simulink model "gm_wlanhdlTimeAndFrequencySynchronization"  (R2025a)
settings: Solver=FixedStepDiscrete  StartTime=0.0  StopTime=stopTime  RelTol=1e-3
InitFcn:
  | wlanFrontEndInit;
undefined symbols (not defined in the file or in its folder): a, b, c, Hd, wlanConfig
libraries: simulink x95, hdlsllib x16, hdlmdlgenlib x12, dspsrcs4 x3, dspsigops x3, dsphdlsigops2 x2, dsphdlfiltering2 x2
(part 11 of 11)

== system gm_wlanhdlTimeAndFrequencySynchronization/WLANTimeAndFrequencySynchronization/Coarse Time Sync/Energy Calculator/magnitudeSquared/MagnitudeSquared ==
  dataIn : Inport  OutDataTypeStr=fixdt(1, 16, 12)  PortDimensions=1  SampleTime=5e-08
      settings: SignalType=complex
  validIn : Inport  Port=2  OutDataTypeStr=boolean  PortDimensions=1  SampleTime=5e-08
  Add : Sum  OutDataTypeStr=fixdt(1, 33, 24)  AccumDataTypeStr=fixdt(1, 33, 24)  SampleTime=6.25e-09
  Complex to Real-Imag : ComplexToRealImag  SampleTime=5e-08
  DTadjust : Subsystem
  Delay1 : Delay  DelayLength=double(2)  InitialCondition=0  SampleTime=5e-08
  Delay3 : Delay  DelayLength=double(2)  InitialCondition=0  SampleTime=5e-08
  Delay4 : RateTransition  InitialCondition=double(0)  OutPortSampleTimeOpt=Multiple of input port sample time  OutPortSampleTimeMultiple=8
  Delay4_absorbed : Delay  DelayLength=0
  Delay5 : RateTransition  InitialCondition=double(0)  OutPortSampleTimeOpt=Multiple of input port sample time  OutPortSampleTimeMultiple=8
  Delay5_absorbed : Delay  DelayLength=0
  Delay6 : Delay  DelayLength=double(2)  InitialCondition=0  SampleTime=5e-08
  Delay61 : RateTransition  InitialCondition=double(0)  OutPortSampleTimeOpt=Multiple of input port sample time  OutPortSampleTimeMultiple=8
  HwModeRegister{,1..3} (4 alike) : Delay  DelayLength=double(1)  InitialCondition=0  SampleTime=6.25e-09
  PipelineRegister : Delay  DelayLength=double(1)  InitialCondition=0  SampleTime=6.25e-09
  PipelineRegister1 : Delay  DelayLength=double(1)  InitialCondition=0  SampleTime=6.25e-09
  Product1 : Product  Inputs=**  OutDataTypeStr=fixdt(1, 32, 24)  SampleTime=6.25e-09
  Product4 : Product  Inputs=**  OutDataTypeStr=fixdt(1, 32, 24)  SampleTime=6.25e-09
  crp_out_delay : Delay  DelayLength=double(1)  InitialCondition=0  SampleTime=6.25e-09
  crp_out_delay1 : Delay  DelayLength=double(1)  InitialCondition=0  SampleTime=6.25e-09
  crp_out_delay2 : Delay  DelayLength=double(1)  InitialCondition=0  SampleTime=6.25e-09
  in0_repeat : RateTransition  Integrity=off  Deterministic=off  OutPortSampleTimeOpt=Multiple of input port sample time  OutPortSampleTimeMultiple=1/8
  in0_repeat1 : RateTransition  Integrity=off  Deterministic=off  OutPortSampleTimeOpt=Multiple of input port sample time  OutPortSampleTimeMultiple=1/8
  in1_repeat : RateTransition  Integrity=off  Deterministic=off  OutPortSampleTimeOpt=Multiple of input port sample time  OutPortSampleTimeMultiple=1/8
  in1_repeat1 : RateTransition  Integrity=off  Deterministic=off  OutPortSampleTimeOpt=Multiple of input port sample time  OutPortSampleTimeMultiple=1/8
  in2_repeat : RateTransition  Integrity=off  Deterministic=off  OutPortSampleTimeOpt=Multiple of input port sample time  OutPortSampleTimeMultiple=1/8
  in2_repeat1 : RateTransition  Integrity=off  Deterministic=off  OutPortSampleTimeOpt=Multiple of input port sample time  OutPortSampleTimeMultiple=1/8
  in3_repeat : RateTransition  Integrity=off  Deterministic=off  OutPortSampleTimeOpt=Multiple of input port sample time  OutPortSampleTimeMultiple=1/8
  rd_{0..4,11} (6 alike) : Delay  DelayLength=double(1)  InitialCondition=0  SampleTime=6.25e-09
  dataOut : Outport  SampleTime=6.25e-09  VectorParamsAs1DForOutWhenUnconnected=off
  validOut : Outport  Port=2  SampleTime=5e-08  VectorParamsAs1DForOutWhenUnconnected=off
  wires:
  DTadjust/1(out) -> dataOut/1
  rd_2/1 -> Add/2
  rd_1/1 -> Add/1
  in1_repeat/1 -> rd_1/1
  Delay5_absorbed/1 -> in2_repeat/1
  Delay4_absorbed/1 -> in1_repeat/1
  in3_repeat/1 -> rd_4/1
  in2_repeat/1 -> rd_2/1
  Delay61/1 -> Delay6/1
  in1_repeat1/1 -> rd_11/1
  rd_3/1 -> HwModeRegister2/1
  in0_repeat1/1 -> rd_0/1
  crp_out_delay/1 -> Delay61/1
  dataIn/1 -> Complex to Real-Imag/1
  Complex to Real-Imag/2 -> Delay3/1
  rd_4/1 -> HwModeRegister3/1
  Delay4/1 -> Delay4_absorbed/1
  rd_0/1 -> HwModeRegister/1
  validIn/1 -> in0_repeat/1
  Delay1/1 -> in1_repeat1/1, in0_repeat1/1
  HwModeRegister/1 -> Product4/1
  Product1/1 -> PipelineRegister1/1
  in0_repeat/1 -> crp_out_delay/1
  Delay6/1 -> validOut/1
  Complex to Real-Imag/1 -> Delay1/1
  rd_11/1 -> HwModeRegister1/1
  HwModeRegister1/1 -> Product4/2
  HwModeRegister2/1 -> Product1/1
  HwModeRegister3/1 -> Product1/2
  Delay3/1 -> in2_repeat1/1, in3_repeat/1
  Product4/1 -> PipelineRegister/1
  PipelineRegister/1 -> crp_out_delay1/1
  Delay5/1 -> Delay5_absorbed/1
  in2_repeat1/1 -> rd_3/1
  crp_out_delay2/1 -> Delay5/1
  PipelineRegister1/1 -> crp_out_delay2/1
  Add/1 -> DTadjust/1(in)
  crp_out_delay1/1 -> Delay4/1

== system gm_wlanhdlTimeAndFrequencySynchronization/WLANTimeAndFrequencySynchronization/Coarse Time Sync/Energy Calculator/magnitudeSquared/MagnitudeSquared1 ==
  dataIn : Inport  OutDataTypeStr=fixdt(1, 35, 27)  PortDimensions=1  SampleTime=6.25e-09
  validIn : Inport  Port=2  OutDataTypeStr=boolean  PortDimensions=1  SampleTime=5e-08
  Add : Sum  OutDataTypeStr=fixdt(1, 71, 54)  AccumDataTypeStr=fixdt(1, 71, 54)  SampleTime=6.25e-09
  Complex to Real-Imag : ComplexToRealImag  SampleTime=6.25e-09
  Delay{,1..3} (4 alike) : Delay  DelayLength=double(1)  InitialCondition=0  SampleTime=5e-08
  Delay{4..5,11,21,31,41,61} (7 alike) : RateTransition  InitialCondition=double(0)  OutPortSampleTimeOpt=Multiple of input port sample time  OutPortSampleTimeMultiple=8
  Delay4_absorbed : Delay  DelayLength=0
  Delay5_absorbed : Delay  DelayLength=0
  Delay6 : Delay  DelayLength=double(3)  InitialCondition=0  SampleTime=5e-08
  HwModeRegister{,1..3} (4 alike) : Delay  DelayLength=double(1)  InitialCondition=0  SampleTime=6.25e-09
  PipelineRegister : Delay  DelayLength=double(1)  InitialCondition=0  SampleTime=6.25e-09
  PipelineRegister1 : Delay  DelayLength=double(1)  InitialCondition=0  SampleTime=6.25e-09
  Product1 : Product  Inputs=**  OutDataTypeStr=fixdt(1, 70, 54)  SampleTime=6.25e-09
  Product4 : Product  Inputs=**  OutDataTypeStr=fixdt(1, 70, 54)  SampleTime=6.25e-09
  crp_out_delay{,1..3} (4 alike) : Delay  DelayLength=double(1)  InitialCondition=0  SampleTime=6.25e-09
  in0_repeat : RateTransition  Integrity=off  Deterministic=off  OutPortSampleTimeOpt=Multiple of input port sample time  OutPortSampleTimeMultiple=1/8
  in0_repeat1 : RateTransition  Integrity=off  Deterministic=off  OutPortSampleTimeOpt=Multiple of input port sample time  OutPortSampleTimeMultiple=1/8
  in1_repeat : RateTransition  Integrity=off  Deterministic=off  OutPortSampleTimeOpt=Multiple of input port sample time  OutPortSampleTimeMultiple=1/8
  in1_repeat1 : RateTransition  Integrity=off  Deterministic=off  OutPortSampleTimeOpt=Multiple of input port sample time  OutPortSampleTimeMultiple=1/8
  in2_repeat : RateTransition  Integrity=off  Deterministic=off  OutPortSampleTimeOpt=Multiple of input port sample time  OutPortSampleTimeMultiple=1/8
  in2_repeat1 : RateTransition  Integrity=off  Deterministic=off  OutPortSampleTimeOpt=Multiple of input port sample time  OutPortSampleTimeMultiple=1/8
  in3_repeat : RateTransition  Integrity=off  Deterministic=off  OutPortSampleTimeOpt=Multiple of input port sample time  OutPortSampleTimeMultiple=1/8
  rd_{0..4,11} (6 alike) : Delay  DelayLength=double(1)  InitialCondition=0  SampleTime=6.25e-09
  dataOut : Outport  SampleTime=6.25e-09  VectorParamsAs1DForOutWhenUnconnected=off
  validOut : Outport  Port=2  SampleTime=5e-08  VectorParamsAs1DForOutWhenUnconnected=off
  wires:
  rd_2/1 -> Add/2
  in2_repeat/1 -> rd_2/1
  in1_repeat/1 -> rd_1/1
  Delay5_absorbed/1 -> in2_repeat/1
  Delay4_absorbed/1 -> in1_repeat/1
  crp_out_delay1/1 -> Delay5/1
  crp_out_delay/1 -> Delay41/1
  PipelineRegister1/1 -> crp_out_delay1/1
  PipelineRegister/1 -> crp_out_delay/1
  Delay31/1 -> Delay3/1
  in0_repeat/1 -> Delay61/1
  Delay11/1 -> Delay1/1
  HwModeRegister1/1 -> Product4/2
  crp_out_delay3/1 -> Delay21/1, Delay31/1
  Delay5/1 -> Delay5_absorbed/1
  crp_out_delay2/1 -> Delay4/1, Delay11/1
  Delay21/1 -> Delay2/1
  Delay61/1 -> Delay6/1
  HwModeRegister2/1 -> Product1/1
  Complex to Real-Imag/2 -> crp_out_delay3/1
  Product4/1 -> PipelineRegister/1
  Complex to Real-Imag/1 -> crp_out_delay2/1
  Delay4/1 -> Delay/1
  rd_3/1 -> HwModeRegister2/1
  Delay6/1 -> validOut/1
  Delay41/1 -> Delay4_absorbed/1
  rd_11/1 -> HwModeRegister1/1
  rd_1/1 -> Add/1
  validIn/1 -> in0_repeat/1
  rd_4/1 -> HwModeRegister3/1
  Delay3/1 -> in3_repeat/1
  dataIn/1 -> Complex to Real-Imag/1
  Delay/1 -> in1_repeat1/1
  Delay2/1 -> in2_repeat1/1
  Product1/1 -> PipelineRegister1/1
  in0_repeat1/1 -> rd_0/1
  Delay1/1 -> in0_repeat1/1
  in1_repeat1/1 -> rd_11/1
  in3_repeat/1 -> rd_4/1
  Add/1 -> dataOut/1
  rd_0/1 -> HwModeRegister/1
  in2_repeat1/1 -> rd_3/1
  HwModeRegister/1 -> Product4/1
  HwModeRegister3/1 -> Product1/2

== system gm_wlanhdlTimeAndFrequencySynchronization/WLANTimeAndFrequencySynchronization/Coarse Time Sync/Energy Calculator/magnitudeSquared/MovingSum ==
  dataIn : Inport  OutDataTypeStr=fixdt(1, 34, 27)  PortDimensions=1  SampleTime=6.25e-09
  validIn : Inport  Port=2  OutDataTypeStr=boolean  PortDimensions=1  SampleTime=5e-08
  Add : Sum  Inputs=+-  OutDataTypeStr=fixdt(1, 35, 27)  AccumDataTypeStr=fixdt(1, 35, 27)  SampleTime=6.25e-09
  Add1 : Sum  OutDataTypeStr=fixdt(1, 35, 27)  AccumDataTypeStr=fixdt(1, 35, 27)  SampleTime=6.25e-09
  Delay12 : RateTransition  InitialCondition=double(0)  OutPortSampleTimeOpt=Multiple of input port sample time  OutPortSampleTimeMultiple=8
  Delay12_absorbed : Delay  DelayLength=0
  Delay{3..6} (4 alike) : Delay  DelayLength=double(1)  InitialCondition=0  SampleTime=5e-08
  Delay31 : RateTransition  InitialCondition=double(0)  OutPortSampleTimeOpt=Multiple of input port sample time  OutPortSampleTimeMultiple=8
  Delay41 : RateTransition  InitialCondition=double(0)  OutPortSampleTimeOpt=Multiple of input port sample time  OutPortSampleTimeMultiple=8
  Delay_Switch : Switch  Criteria=u2 ~= 0  Threshold=double(0)  OutDataTypeStr=fixdt(1, 35, 27)  SampleTime=6.25e-09  SaturateOnIntegerOverflow=off  InputSameDT=off
  Shift Arithmetic : ArithShift  BitShiftNumber=double(1)  BinPtShiftNumber=double(0)
  "Synchronous Enabled 16 Sample Delay " : Subsystem
  Synchronous Enabled Unit Delay_lowered : RateTransition  InitialCondition=double(0)  OutPortSampleTimeOpt=Multiple of input port sample time  OutPortSampleTimeMultiple=8
  Synchronous Enabled Unit Delay_lowered_absorbed : Delay  DelayLength=0
  crp_out_delay : Delay  DelayLength=double(1)  InitialCondition=0  SampleTime=6.25e-09
  crp_out_delay1 : Delay  DelayLength=double(1)  InitialCondition=0  SampleTime=6.25e-09
  in0_repeat : RateTransition  Integrity=off  Deterministic=off  OutPortSampleTimeOpt=Multiple of input port sample time  OutPortSampleTimeMultiple=1/8
  in0_repeat1 : RateTransition  Integrity=off  Deterministic=off  OutPortSampleTimeOpt=Multiple of input port sample time  OutPortSampleTimeMultiple=1/8
  in1_repeat : RateTransition  Integrity=off  Deterministic=off  OutPortSampleTimeOpt=Multiple of input port sample time  OutPortSampleTimeMultiple=1/8
  in2_repeat : RateTransition  Integrity=off  Deterministic=off  OutPortSampleTimeOpt=Multiple of input port sample time  OutPortSampleTimeMultiple=1/8
  in2_repeat1 : RateTransition  Integrity=off  Deterministic=off  OutPortSampleTimeOpt=Multiple of input port sample time  OutPortSampleTimeMultiple=1/8
  rd_{1,3,5,11,21,31} (6 alike) : Delay  DelayLength=double(1)  InitialCondition=0  SampleTime=6.25e-09
  rd_2 : Delay  DelayLength=double(3)  InitialCondition=0  SampleTime=6.25e-09
  rd_4 : Delay  DelayLength=double(2)  InitialCondition=0  SampleTime=6.25e-09
  dataOut : Outport  SampleTime=5e-08  VectorParamsAs1DForOutWhenUnconnected=off
  validOut : Outport  Port=2  SampleTime=5e-08  VectorParamsAs1DForOutWhenUnconnected=off
  wires:
  rd_21/1 -> Add1/2, rd_5/1
  rd_11/1 -> Add1/1
  Delay41/1 -> Delay4/1
  Delay6/1 -> validOut/1
  in0_repeat1/1 -> Delay41/1, rd_4/1
  rd_2/1 -> Add/2
  in1_repeat/1 -> rd_21/1
  Delay3/1 -> in0_repeat1/1
  in2_repeat/1 -> rd_2/1
  rd_1/1 -> Add/1
  Delay31/1 -> Delay3/1
  dataIn/1 -> "Synchronous Enabled 16 Sample Delay "/1(dataIn), rd_1/1
  in0_repeat/1 -> Delay31/1
  rd_3/1 -> Shift Arithmetic/1
  "Synchronous Enabled 16 Sample Delay "/1(dataOut) -> in2_repeat/1
  validIn/1 -> "Synchronous Enabled 16 Sample Delay "/2(en), in0_repeat/1
  Synchronous Enabled Unit Delay_lowered_absorbed/1 -> in1_repeat/1, Delay5/1
  rd_5/1 -> Delay_Switch/3
  rd_4/1 -> Delay_Switch/2
  crp_out_delay/1 -> Delay12/1
  crp_out_delay1/1 -> Synchronous Enabled Unit Delay_lowered/1
  Synchronous Enabled Unit Delay_lowered/1 -> Synchronous Enabled Unit Delay_lowered_absorbed/1
  rd_31/1 -> Delay_Switch/1
  Delay4/1 -> Delay6/1
  Shift Arithmetic/1 -> crp_out_delay/1
  Delay_Switch/1 -> crp_out_delay1/1
  Add1/1 -> rd_31/1
  Add/1 -> rd_3/1
  Delay12/1 -> Delay12_absorbed/1
  in2_repeat1/1 -> rd_11/1
  Delay12_absorbed/1 -> in2_repeat1/1
  Delay5/1 -> dataOut/1

== system gm_wlanhdlTimeAndFrequencySynchronization/WLANTimeAndFrequencySynchronization/Coarse Time Sync/Energy Calculator/streamSynchronizer/StreamSyncronizer ==
  pop : Inport  OutDataTypeStr=boolean  PortDimensions=1  SampleTime=5e-08
  dataIn : Inport  Port=2  OutDataTypeStr=fixdt(1, 71, 54)  PortDimensions=1  SampleTime=5e-08
  push : Inport  Port=3  OutDataTypeStr=boolean  PortDimensions=1  SampleTime=5e-08
  StreamSyncronizer : MATLAB Function  InitFcn=Simulink.suppressDiagnostic(gcb, 'Stateflow:Runtime:DataOverflowErrorMSLD');  TreatAsAtomicUnit=on  mask{depth=256}
      mask help: Synchronize two data streams with a FIFO.
  dataOut : Outport  SampleTime=5e-08  VectorParamsAs1DForOutWhenUnconnected=off
  validOut : Outport  Port=2  SampleTime=5e-08  VectorParamsAs1DForOutWhenUnconnected=off
  wires:
  StreamSyncronizer/2(validOut) -> validOut/1
  StreamSyncronizer/1(dataOut) -> dataOut/1
  push/1 -> StreamSyncronizer/3(push)
  dataIn/1 -> StreamSyncronizer/2(dataIn)
  pop/1 -> StreamSyncronizer/1(pop)

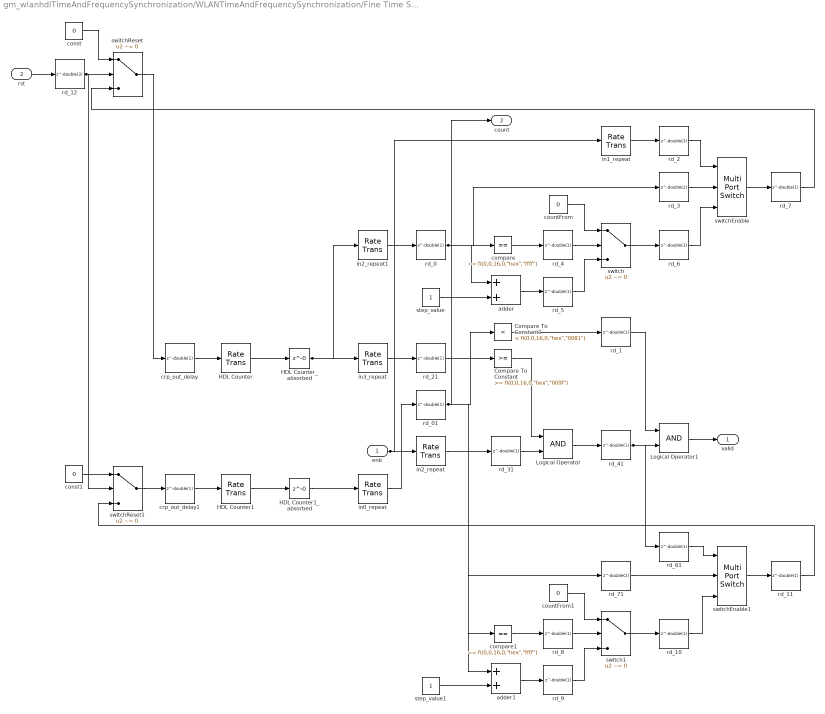
== system gm_wlanhdlTimeAndFrequencySynchronization/WLANTimeAndFrequencySynchronization/Fine Time Sync/Peak Searcher/maxPeakSearcher/extractLTFs ==
  enb : Inport  OutDataTypeStr=boolean  PortDimensions=1  SampleTime=5e-08
  rst : Inport  Port=2  OutDataTypeStr=boolean  PortDimensions=1  SampleTime=6.25e-09
  Compare To Constant : simulink/Logic and Bit Operations/Compare To Constant  relop=>=  const="fi(0,0,16,0,\"hex\",\"009f\")"  OutDataTypeStr=boolean
  Compare To Constant1 : simulink/Logic and Bit Operations/Compare To Constant  relop=<  const="fi(0,0,16,0,\"hex\",\"0081\")"  OutDataTypeStr=boolean
  HDL Counter : RateTransition  InitialCondition=double(0)  OutPortSampleTimeOpt=Multiple of input port sample time  OutPortSampleTimeMultiple=8
  HDL Counter1 : RateTransition  InitialCondition=double(0)  OutPortSampleTimeOpt=Multiple of input port sample time  OutPortSampleTimeMultiple=8
  HDL Counter1_absorbed : Delay  DelayLength=0
  HDL Counter_absorbed : Delay  DelayLength=0
  Logical Operator : Logic  AllPortsSameDT=off  OutDataTypeStr=boolean  SampleTime=6.25e-09
  Logical Operator1 : Logic  AllPortsSameDT=off  OutDataTypeStr=boolean  SampleTime=6.25e-09
  adder : Sum  OutDataTypeStr=uint16  AccumDataTypeStr=uint16  SampleTime=6.25e-09
  adder1 : Sum  OutDataTypeStr=uint16  AccumDataTypeStr=uint16  SampleTime=6.25e-09
  compare : simulink/Logic and Bit Operations/Compare To Constant  relop===  const="fi(0,0,16,0,\"hex\",\"ffff\")"  OutDataTypeStr=boolean
  compare1 : simulink/Logic and Bit Operations/Compare To Constant  relop===  const="fi(0,0,16,0,\"hex\",\"ffff\")"  OutDataTypeStr=boolean
  const : Constant  Value=0  VectorParams1D=off  OutDataTypeStr=uint16  SampleTime=6.25e-09
  const1 : Constant  Value=0  VectorParams1D=off  OutDataTypeStr=uint16  SampleTime=6.25e-09
  countFrom : Constant  Value=0  VectorParams1D=off  OutDataTypeStr=uint16  SampleTime=6.25e-09
  countFrom1 : Constant  Value=0  VectorParams1D=off  OutDataTypeStr=uint16  SampleTime=6.25e-09
  crp_out_delay : Delay  DelayLength=double(1)  InitialCondition=0  SampleTime=6.25e-09
  crp_out_delay1 : Delay  DelayLength=double(1)  InitialCondition=0  SampleTime=6.25e-09
  in0_repeat : RateTransition  Integrity=off  Deterministic=off  OutPortSampleTimeOpt=Multiple of input port sample time  OutPortSampleTimeMultiple=1/8
  in1_repeat : RateTransition  Integrity=off  Deterministic=off  OutPortSampleTimeOpt=Multiple of input port sample time  OutPortSampleTimeMultiple=1/8
  in2_repeat : RateTransition  Integrity=off  Deterministic=off  OutPortSampleTimeOpt=Multiple of input port sample time  OutPortSampleTimeMultiple=1/8
  in2_repeat1 : RateTransition  Integrity=off  Deterministic=off  OutPortSampleTimeOpt=Multiple of input port sample time  OutPortSampleTimeMultiple=1/8
  in3_repeat : RateTransition  Integrity=off  Deterministic=off  OutPortSampleTimeOpt=Multiple of input port sample time  OutPortSampleTimeMultiple=1/8
  rd_{0..1,4..11,21,31,41,61} (14 alike) : Delay  DelayLength=double(1)  InitialCondition=0  SampleTime=6.25e-09
  rd_01 : Delay  DelayLength=double(1)  InitialCondition=0  SampleTime=6.25e-09
  rd_12 : Delay  DelayLength=double(3)  InitialCondition=0  SampleTime=6.25e-09
  rd_2 : Delay  DelayLength=double(3)  InitialCondition=0  SampleTime=6.25e-09
  rd_3 : Delay  DelayLength=double(2)  InitialCondition=0  SampleTime=6.25e-09
  rd_71 : Delay  DelayLength=double(2)  InitialCondition=0  SampleTime=6.25e-09
  step_value : Constant  VectorParams1D=off  OutDataTypeStr=uint16  SampleTime=6.25e-09
  step_value1 : Constant  VectorParams1D=off  OutDataTypeStr=uint16  SampleTime=6.25e-09
  switch : Switch  Criteria=u2 ~= 0  Threshold="fi(0,0,1,0,\"hex\",\"0\")"  OutDataTypeStr=uint16  SampleTime=6.25e-09  SaturateOnIntegerOverflow=off  InputSameDT=off
  switch1 : Switch  Criteria=u2 ~= 0  Threshold="fi(0,0,1,0,\"hex\",\"0\")"  OutDataTypeStr=uint16  SampleTime=6.25e-09  SaturateOnIntegerOverflow=off  InputSameDT=off
  switchEnable : MultiPortSwitch  DataPortOrder=Zero-based contiguous  Inputs=2  DiagnosticForDefault=None  zeroidx=on  OutDataTypeStr=uint16  SampleTime=6.25e-09  SaturateOnIntegerOverflow=off  InputSameDT=off
  switchEnable1 : MultiPortSwitch  DataPortOrder=Zero-based contiguous  Inputs=2  DiagnosticForDefault=None  zeroidx=on  OutDataTypeStr=uint16  SampleTime=6.25e-09  SaturateOnIntegerOverflow=off  InputSameDT=off
  switchReset : Switch  Criteria=u2 ~= 0  Threshold="fi(0,0,1,0,\"hex\",\"0\")"  OutDataTypeStr=uint16  SampleTime=6.25e-09  SaturateOnIntegerOverflow=off  InputSameDT=off
  switchReset1 : Switch  Criteria=u2 ~= 0  Threshold="fi(0,0,1,0,\"hex\",\"0\")"  OutDataTypeStr=uint16  SampleTime=6.25e-09  SaturateOnIntegerOverflow=off  InputSameDT=off
  valid : Outport  SampleTime=6.25e-09
  count : Outport  Port=2  SampleTime=6.25e-09
  wires:
  rd_7/1 -> switchReset/3
  rd_10/1 -> switchEnable1/3
  rd_61/1 -> switchEnable1/1
  rd_6/1 -> switchEnable/3
  rd_71/1 -> switchEnable1/2
  rd_41/1 -> rd_61/1, Logical Operator1/2
  switch/1 -> rd_6/1
  countFrom1/1 -> switch1/1
  switchEnable1/1 -> rd_11/1
  Logical Operator/1 -> rd_41/1
  rd_11/1 -> switchReset1/3
  rd_5/1 -> switch/3
  rd_4/1 -> switch/2
  countFrom/1 -> switch/1
  rd_3/1 -> switchEnable/2
  HDL Counter1_absorbed/1 -> in0_repeat/1
  in1_repeat/1 -> rd_2/1
  in2_repeat/1 -> rd_31/1
  compare1/1 -> rd_8/1
  crp_out_delay1/1 -> HDL Counter1/1
  crp_out_delay/1 -> HDL Counter/1
  switchReset1/1 -> crp_out_delay1/1
  HDL Counter/1 -> HDL Counter_absorbed/1
  rd_31/1 -> Logical Operator/2
  const1/1 -> switchReset1/1
  HDL Counter_absorbed/1 -> in2_repeat1/1, in3_repeat/1
  rd_12/1 -> switchReset1/2, switchReset/2
  switchEnable/1 -> rd_7/1
  switchReset/1 -> crp_out_delay/1
  const/1 -> switchReset/1
  step_value/1 -> adder/2
  rd_9/1 -> switch1/3
  in3_repeat/1 -> rd_21/1
  enb/1 -> in2_repeat/1, in1_repeat/1
  Logical Operator1/1 -> valid/1
  in0_repeat/1 -> rd_01/1
  compare/1 -> rd_4/1
  rd_0/1 -> compare/1, adder/1, rd_3/1
  rd_21/1 -> Compare To Constant/1
  rst/1 -> rd_12/1
  rd_01/1 -> count/1, rd_71/1, Compare To Constant1/1, compare1/1, adder1/1
  switch1/1 -> rd_10/1
  step_value1/1 -> adder1/2
  Compare To Constant/1 -> Logical Operator/1
  HDL Counter1/1 -> HDL Counter1_absorbed/1
  adder/1 -> rd_5/1
  rd_2/1 -> switchEnable/1
  rd_1/1 -> Logical Operator1/1
  Compare To Constant1/1 -> rd_1/1
  rd_8/1 -> switch1/2
  in2_repeat1/1 -> rd_0/1
  adder1/1 -> rd_9/1

== system gm_wlanhdlTimeAndFrequencySynchronization/WLANTimeAndFrequencySynchronization/Fine Time Sync/Peak Searcher/maxPeakSearcher/maxPeakSearcher ==
  dataIn : Inport  OutDataTypeStr=fixdt(1, 32, 15)  PortDimensions=1  SampleTime=5e-08
  validIn : Inport  Port=2  OutDataTypeStr=boolean  PortDimensions=1  SampleTime=5e-08
  countValue : Inport  Port=3  OutDataTypeStr=uint16  PortDimensions=1  SampleTime=5e-08
  reset : Inport  Port=4  OutDataTypeStr=boolean  PortDimensions=1  SampleTime=5e-08
  maxPeakSearcher : MATLAB Function  TreatAsAtomicUnit=on
  maxPeak : Outport  SampleTime=5e-08  VectorParamsAs1DForOutWhenUnconnected=off
  wires:
  maxPeakSearcher/1(maxPeak) -> maxPeak/1
  reset/1 -> maxPeakSearcher/4(reset)
  countValue/1 -> maxPeakSearcher/3(countValue)
  validIn/1 -> maxPeakSearcher/2(validIn)
  dataIn/1 -> maxPeakSearcher/1(dataIn)

== system gm_wlanhdlTimeAndFrequencySynchronization/WLANTimeAndFrequencySynchronization/Fine Time Sync/Peak Searcher/peakDetector/dataSelector  ==
  syncEn : Inport  OutDataTypeStr=boolean  PortDimensions=1  SampleTime=5e-08
  dataIn : Inport  Port=2  OutDataTypeStr=fixdt(1, 16, 12)  PortDimensions=1  SampleTime=5e-08
      settings: SignalType=complex
  validIn : Inport  Port=3  OutDataTypeStr=boolean  PortDimensions=1  SampleTime=5e-08
  MATLAB Function1 : MATLAB Function  TreatAsAtomicUnit=on
  dataOut : Outport  SampleTime=5e-08  VectorParamsAs1DForOutWhenUnconnected=off
  wires:
  syncEn/1 -> MATLAB Function1/1(syncEn)
  dataIn/1 -> MATLAB Function1/2(dataIn)
  validIn/1 -> MATLAB Function1/3(validIn)
  MATLAB Function1/1(dataOut) -> dataOut/1

== system gm_wlanhdlTimeAndFrequencySynchronization/WLANTimeAndFrequencySynchronization/Coarse Time Sync/Energy Calculator/magnitudeSquared/MagnitudeSquared/DTadjust ==
  in : Inport  OutDataTypeStr=fixdt(1, 33, 24)  PortDimensions=1  SampleTime=6.25e-09
  DTadjust : MATLAB Function  TreatAsAtomicUnit=on
  out : Outport  SampleTime=6.25e-09  VectorParamsAs1DForOutWhenUnconnected=off
  wires:
  DTadjust/1(out) -> out/1
  in/1 -> DTadjust/1(in)

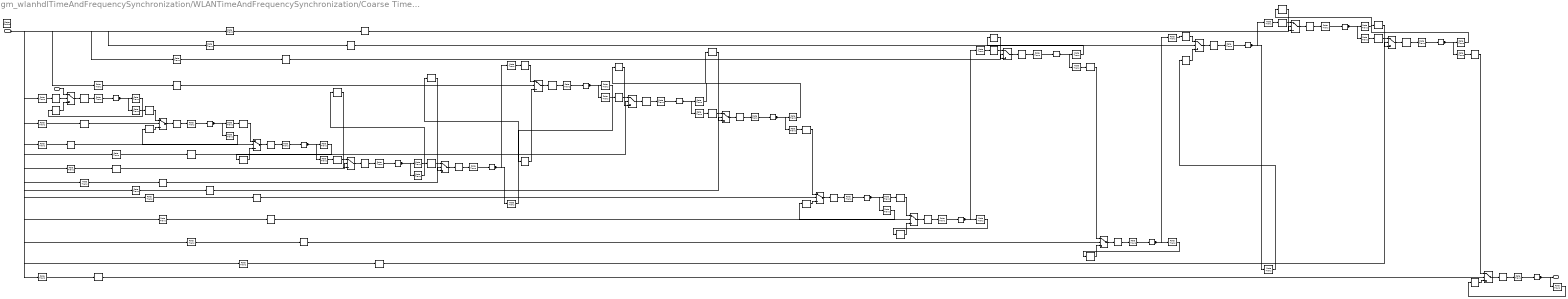
== system gm_wlanhdlTimeAndFrequencySynchronization/WLANTimeAndFrequencySynchronization/Coarse Time Sync/Energy Calculator/magnitudeSquared/MovingSum/Synchronous Enabled 16 Sample Delay  ==
  dataIn : Inport  OutDataTypeStr=fixdt(1, 34, 27)  PortDimensions=1  SampleTime=6.25e-09
  en : Inport  Port=2  OutDataTypeStr=boolean  PortDimensions=1  SampleTime=5e-08
  Delay1_lowered{,1..15} (16 alike) : RateTransition  InitialCondition=double(0)  OutPortSampleTimeOpt=Multiple of input port sample time  OutPortSampleTimeMultiple=8
  Delay1_lowered_absorbed{,1..15} (16 alike) : Delay  DelayLength=0
  Delay_Switch{,1..15} (16 alike) : Switch  Criteria=u2 ~= 0  Threshold=double(0)  OutDataTypeStr=fixdt(1, 34, 27)  SampleTime=6.25e-09  SaturateOnIntegerOverflow=off  InputSameDT=off
  StateControl : StateControl  StateControl=Synchronous
  crp_out_delay{,1..15} (16 alike) : Delay  DelayLength=double(1)  InitialCondition=0  SampleTime=6.25e-09
  in0_repeat{,1..14} (15 alike) : RateTransition  Integrity=off  Deterministic=off  OutPortSampleTimeOpt=Multiple of input port sample time  OutPortSampleTimeMultiple=1/8
  in1_repeat{,1..15} (16 alike) : RateTransition  Integrity=off  Deterministic=off  OutPortSampleTimeOpt=Multiple of input port sample time  OutPortSampleTimeMultiple=1/8
  in2_repeat{,1..15} (16 alike) : RateTransition  Integrity=off  Deterministic=off  OutPortSampleTimeOpt=Multiple of input port sample time  OutPortSampleTimeMultiple=1/8
  rd_0 : Delay  DelayLength=double(2)  InitialCondition=0  SampleTime=6.25e-09
  rd_01 : Delay  DelayLength=double(1)  InitialCondition=0  SampleTime=6.25e-09
  rd_010 : Delay  DelayLength=double(1)  InitialCondition=0  SampleTime=6.25e-09
  rd_011 : Delay  DelayLength=double(1)  InitialCondition=0  SampleTime=6.25e-09
  rd_012 : Delay  DelayLength=double(1)  InitialCondition=0  SampleTime=6.25e-09
  rd_013 : Delay  DelayLength=double(1)  InitialCondition=0  SampleTime=6.25e-09
  rd_014 : Delay  DelayLength=double(1)  InitialCondition=0  SampleTime=6.25e-09
  rd_015 : Delay  DelayLength=double(1)  InitialCondition=0  SampleTime=6.25e-09
  rd_02 : Delay  DelayLength=double(1)  InitialCondition=0  SampleTime=6.25e-09
  rd_03 : Delay  DelayLength=double(1)  InitialCondition=0  SampleTime=6.25e-09
  rd_04 : Delay  DelayLength=double(1)  InitialCondition=0  SampleTime=6.25e-09
  rd_05 : Delay  DelayLength=double(1)  InitialCondition=0  SampleTime=6.25e-09
  rd_06 : Delay  DelayLength=double(1)  InitialCondition=0  SampleTime=6.25e-09
  rd_07 : Delay  DelayLength=double(1)  InitialCondition=0  SampleTime=6.25e-09
  rd_08 : Delay  DelayLength=double(1)  InitialCondition=0  SampleTime=6.25e-09
  rd_09 : Delay  DelayLength=double(1)  InitialCondition=0  SampleTime=6.25e-09
  rd_1 : Delay  DelayLength=double(2)  InitialCondition=0  SampleTime=6.25e-09
  rd_{2,11..19,21..29,110..115,210..214} (30 alike) : Delay  DelayLength=double(1)  InitialCondition=0  SampleTime=6.25e-09
  dataOut : Outport  SampleTime=5e-08  VectorParamsAs1DForOutWhenUnconnected=off
  wires:
  crp_out_delay9/1 -> Delay1_lowered9/1
  crp_out_delay5/1 -> Delay1_lowered5/1
  Delay1_lowered14/1 -> Delay1_lowered_absorbed14/1
  in0_repeat2/1 -> rd_03/1
  Delay1_lowered7/1 -> Delay1_lowered_absorbed7/1
  crp_out_delay3/1 -> Delay1_lowered3/1
  in0_repeat12/1 -> rd_013/1
  Delay_Switch15/1 -> crp_out_delay15/1
  in0_repeat3/1 -> rd_04/1
  crp_out_delay15/1 -> Delay1_lowered15/1
  in0_repeat6/1 -> rd_07/1
  in2_repeat12/1 -> rd_211/1
  Delay_Switch2/1 -> crp_out_delay2/1
  crp_out_delay1/1 -> Delay1_lowered1/1
  Delay_Switch13/1 -> crp_out_delay13/1
  rd_02/1 -> Delay_Switch2/1
  in0_repeat4/1 -> rd_05/1
  in0_repeat5/1 -> rd_06/1
  Delay1_lowered11/1 -> Delay1_lowered_absorbed11/1
  Delay_Switch1/1 -> crp_out_delay1/1
  crp_out_delay10/1 -> Delay1_lowered10/1
  Delay1_lowered4/1 -> Delay1_lowered_absorbed4/1
  in2_repeat2/1 -> rd_21/1
  Delay1_lowered_absorbed7/1 -> in0_repeat7/1, in2_repeat7/1
  Delay1_lowered_absorbed15/1 -> in2_repeat15/1, dataOut/1
  Delay1_lowered8/1 -> Delay1_lowered_absorbed8/1
  in1_repeat3/1 -> rd_13/1
  rd_24/1 -> Delay_Switch5/3
  rd_210/1 -> Delay_Switch11/3
  Delay1_lowered_absorbed3/1 -> in2_repeat3/1, in0_repeat3/1
  Delay1_lowered5/1 -> Delay1_lowered_absorbed5/1
  rd_26/1 -> Delay_Switch7/3
  in2_repeat14/1 -> rd_213/1
  rd_08/1 -> Delay_Switch8/1
  rd_22/1 -> Delay_Switch3/3
  Delay1_lowered13/1 -> Delay1_lowered_absorbed13/1
  dataIn/1 -> Delay_Switch/1
  rd_213/1 -> Delay_Switch14/3
  rd_18/1 -> Delay_Switch8/2
  in1_repeat14/1 -> rd_114/1
  Delay_Switch10/1 -> crp_out_delay10/1
  Delay1_lowered_absorbed14/1 -> in2_repeat14/1, in0_repeat14/1
  rd_27/1 -> Delay_Switch8/3
  rd_0/1 -> Delay_Switch/2
  rd_112/1 -> Delay_Switch12/2
  rd_15/1 -> Delay_Switch5/2
  Delay1_lowered10/1 -> Delay1_lowered_absorbed10/1
  in1_repeat1/1 -> rd_11/1
  in1_repeat13/1 -> rd_113/1
  rd_111/1 -> Delay_Switch11/2
  Delay1_lowered_absorbed5/1 -> in0_repeat5/1, in2_repeat5/1
  in0_repeat8/1 -> rd_09/1
  Delay1_lowered_absorbed1/1 -> in0_repeat1/1, in2_repeat1/1
  rd_12/1 -> Delay_Switch2/2
  Delay1_lowered9/1 -> Delay1_lowered_absorbed9/1
  en/1 -> in1_repeat/1, in1_repeat1/1, in1_repeat4/1, in1_repeat15/1, in1_repeat2/1, in1_repeat13/1, in1_repeat10/1, in1_repeat5/1, in1_repeat3/1, in1_repeat8/1, in1_repeat7/1, in1_repeat11/1, in1_repeat14/1, in1_repeat12/1, in1_repeat6/1, in1_repeat9/1
  rd_011/1 -> Delay_Switch11/1
  in2_repeat/1 -> rd_1/1
  crp_out_delay13/1 -> Delay1_lowered13/1
  in1_repeat5/1 -> rd_15/1
  rd_29/1 -> Delay_Switch10/3
  Delay_Switch8/1 -> crp_out_delay8/1
  rd_14/1 -> Delay_Switch4/2
  Delay1_lowered12/1 -> Delay1_lowered_absorbed12/1
  in1_repeat12/1 -> rd_112/1
  Delay1_lowered6/1 -> Delay1_lowered_absorbed6/1
  rd_110/1 -> Delay_Switch10/2
  in2_repeat3/1 -> rd_22/1
  Delay1_lowered_absorbed2/1 -> in2_repeat2/1, in0_repeat2/1
  in2_repeat1/1 -> rd_2/1
  in2_repeat13/1 -> rd_212/1
  in2_repeat5/1 -> rd_24/1
  rd_21/1 -> Delay_Switch2/3
  crp_out_delay8/1 -> Delay1_lowered8/1
  rd_01/1 -> Delay_Switch1/1
  Delay1_lowered_absorbed9/1 -> in0_repeat9/1, in2_repeat9/1
  in2_repeat9/1 -> rd_28/1
  in1_repeat2/1 -> rd_12/1
  rd_13/1 -> Delay_Switch3/2
  in2_repeat11/1 -> rd_210/1
  Delay_Switch7/1 -> crp_out_delay7/1
  in1_repeat10/1 -> rd_110/1
  in1_repeat9/1 -> rd_19/1
  in1_repeat11/1 -> rd_111/1
  rd_014/1 -> Delay_Switch14/1
  rd_015/1 -> Delay_Switch15/1
  in2_repeat10/1 -> rd_29/1
  in1_repeat4/1 -> rd_14/1
  in1_repeat6/1 -> rd_16/1
  in2_repeat7/1 -> rd_26/1
  rd_05/1 -> Delay_Switch5/1
  crp_out_delay6/1 -> Delay1_lowered6/1
  rd_113/1 -> Delay_Switch13/2
  rd_115/1 -> Delay_Switch15/2
  Delay_Switch9/1 -> crp_out_delay9/1
  in2_repeat8/1 -> rd_27/1
  Delay_Switch3/1 -> crp_out_delay3/1
  rd_17/1 -> Delay_Switch7/2
  crp_out_delay7/1 -> Delay1_lowered7/1
  rd_07/1 -> Delay_Switch7/1
  in0_repeat9/1 -> rd_010/1
  in2_repeat4/1 -> rd_23/1
  in1_repeat15/1 -> rd_115/1
  Delay1_lowered_absorbed4/1 -> in0_repeat4/1, in2_repeat4/1
  in1_repeat7/1 -> rd_17/1
  rd_16/1 -> Delay_Switch6/2
  Delay_Switch6/1 -> crp_out_delay6/1
  in2_repeat15/1 -> rd_214/1
  in1_repeat8/1 -> rd_18/1
  Delay1_lowered_absorbed11/1 -> in0_repeat11/1, in2_repeat11/1
  in1_repeat/1 -> rd_0/1
  crp_out_delay/1 -> Delay1_lowered/1
  in0_repeat13/1 -> rd_014/1
  in0_repeat/1 -> rd_01/1
  crp_out_delay11/1 -> Delay1_lowered11/1
  Delay_Switch14/1 -> crp_out_delay14/1
  rd_25/1 -> Delay_Switch6/3
  rd_212/1 -> Delay_Switch13/3
  Delay1_lowered_absorbed10/1 -> in2_repeat10/1, in0_repeat10/1
  crp_out_delay2/1 -> Delay1_lowered2/1
  Delay1_lowered15/1 -> Delay1_lowered_absorbed15/1
  Delay1_lowered3/1 -> Delay1_lowered_absorbed3/1
  rd_010/1 -> Delay_Switch10/1
  rd_211/1 -> Delay_Switch12/3
  rd_28/1 -> Delay_Switch9/3
  Delay1_lowered2/1 -> Delay1_lowered_absorbed2/1
  Delay1_lowered_absorbed8/1 -> in2_repeat8/1, in0_repeat8/1
  rd_09/1 -> Delay_Switch9/1
  rd_11/1 -> Delay_Switch1/2
  in0_repeat14/1 -> rd_015/1
  in2_repeat6/1 -> rd_25/1
  rd_04/1 -> Delay_Switch4/1
  rd_06/1 -> Delay_Switch6/1
  Delay_Switch5/1 -> crp_out_delay5/1
  Delay1_lowered1/1 -> Delay1_lowered_absorbed1/1
  Delay_Switch4/1 -> crp_out_delay4/1
  rd_012/1 -> Delay_Switch12/1
  rd_114/1 -> Delay_Switch14/2
  Delay1_lowered_absorbed6/1 -> in0_repeat6/1, in2_repeat6/1
  rd_1/1 -> Delay_Switch/3
  Delay1_lowered_absorbed13/1 -> in0_repeat13/1, in2_repeat13/1
  rd_03/1 -> Delay_Switch3/1
  Delay1_lowered/1 -> Delay1_lowered_absorbed/1
  rd_23/1 -> Delay_Switch4/3
  Delay_Switch11/1 -> crp_out_delay11/1
  rd_214/1 -> Delay_Switch15/3
  Delay1_lowered_absorbed/1 -> in0_repeat/1, in2_repeat/1
  rd_19/1 -> Delay_Switch9/2
  crp_out_delay12/1 -> Delay1_lowered12/1
  Delay_Switch12/1 -> crp_out_delay12/1
  crp_out_delay4/1 -> Delay1_lowered4/1
  in0_repeat7/1 -> rd_08/1
  in0_repeat1/1 -> rd_02/1
  Delay_Switch/1 -> crp_out_delay/1
  Delay1_lowered_absorbed12/1 -> in2_repeat12/1, in0_repeat12/1
  in0_repeat10/1 -> rd_011/1
  rd_2/1 -> Delay_Switch1/3
  crp_out_delay14/1 -> Delay1_lowered14/1
  rd_013/1 -> Delay_Switch13/1
  in0_repeat11/1 -> rd_012/1

== matlab function gm_wlanhdlTimeAndFrequencySynchronization/WLANTimeAndFrequencySynchronization/Coarse Time Sync/Peak Detector/searchStartOfFrame/searchStartOfFrame ==
  data: thresholdValid input; valid input; syncOut output; wlanConfig parameter
function syncOut  = searchStartOfFrame(thresholdValid,valid,wlanConfig)
%#codegen
persistent countVal;
persistent countEnb;
persistent validCount;
persistent detectFlag;
persistent detectFlagCount;

WL = ceil(log2(wlanConfig.lstfLen*10));
if isempty(countVal)
    countVal = fi(0,0,WL,0);
    countEnb = false;
end
if isempty(detectFlag)
    detectFlag = false;
    detectFlagCount = fi(0,0,WL,0);
end
if isempty(validCount)
    validCount = fi(0,0,WL,0); % Considering max count of 10 for STFs
end
if valid && thresholdValid 
    validCount(:) = validCount + 1;
    countEnb = true;
end
if detectFlagCount > 0
    detectFlagCount(:) = detectFlagCount+1;
end
if countEnb
    countVal(:) = countVal + 1;
    if countVal == wlanConfig.lstfLen*10+1
        countVal(:) = 0;
        countEnb = false;
        if validCount > wlanConfig.lstfLen*5
            detectFlag = true;
            detectFlagCount(:) =1;
        else
            detectFlag = false;
        end
        validCount(:) = 0;
    end
end

if detectFlagCount > wlanConfig.lstfLen*10
    detectFlagCount(:)=0;
    detectFlag = false;
end
syncOut = detectFlag;

== matlab function gm_wlanhdlTimeAndFrequencySynchronization/WLANTimeAndFrequencySynchronization/Coarse Time Sync/Stream Synchronizer/StreamSyncronizer/StreamSyncronizer ==
  data: pop input; dataIn input; dataOut output; push input; validOut output; depth parameter
function [dataOut, validOut] = SynchronousFIFO(pop,dataIn,push,depth)
    %#codegen
    
    coder.extrinsic('warning');
    coder.extrinsic('num2str');
    
    persistent wrAddr rdAddr dataOutReg validOutReg mem mem1 mem2 level;
    
    %------------------------------------------------------------------------
    % Constants
    %------------------------------------------------------------------------
    
    addrWL = nextpow2(depth);
    
    %------------------------------------------------------------------------
    % Persistent variable initialization
    %------------------------------------------------------------------------
    
    if isempty(mem)
        
        wrAddr      = fi(0,0,addrWL,0,hdlfimath);
        rdAddr      = fi(0,0,addrWL,0,hdlfimath);
        dataOutReg  = cast(0,'like',dataIn);
        validOutReg = false;
        mem         = zeros(depth,1,'like',dataIn);
        mem1         = zeros(depth,1,'like',dataIn);
        mem2         = zeros(depth,1,'like',dataIn);
        % For generating warnings only. Not for code gen.
        level       = int16(0);
                
    end
    
    %------------------------------------------------------------------------
    % Outputs
    %------------------------------------------------------------------------
    
    dataOut  = dataOutReg;
    validOut = validOutReg;
    
    %------------------------------------------------------------------------
    % Calculate next state values
    %------------------------------------------------------------------------
    
    if pop
        
        dataOutReg(:) = mem(rdAddr+1);
        rdAddr(:)     = rdAddr+1;
        level(:)      = level-1;
        
        if level < 0
            warning('Buffer underflow: attempt to pop data out of empty buffer.');
        end
        
    end
    
    if push
        
        mem(wrAddr+1) = dataIn;
        wrAddr(:)     = wrAddr+1;
        level(:)      = level+1;
        
        if level > depth            
            warning(['Buffer overflow: attempt to push data into full buffer. Level = ', num2str(level), '.']);
        end
        
    end
    
    validOutReg = pop;
    
end

== matlab function gm_wlanhdlTimeAndFrequencySynchronization/WLANTimeAndFrequencySynchronization/Rx Filter/DTConverter/DTConverter ==
  data: dataIn1 input; dataOut output; dataIn2 input
function dataOut = DTConverter(dataIn1,dataIn2)
%#codegen
dataOut = cast(dataIn2,'like',dataIn1);
end

== matlab function gm_wlanhdlTimeAndFrequencySynchronization/WLANTimeAndFrequencySynchronization/Coarse CFO Estimation and Correction/Coarse CFO Correction/DTConverter/DTConverter ==
  data: dataIn1 input; dataOut output; dataIn2 input
function dataOut = DTConverter(dataIn1,dataIn2)
%#codegen
dataOut = cast(dataIn2,'like',dataIn1);
end

== matlab function gm_wlanhdlTimeAndFrequencySynchronization/WLANTimeAndFrequencySynchronization/Fine CFO Estimation and Correction/Fine CFO Correction/DTConverter/DTConverter ==
  data: dataIn1 input; dataOut output; dataIn2 input
function dataOut = DTConverter(dataIn1,dataIn2)
%#codegen
dataOut = cast(dataIn2,'like',dataIn1);
end

== matlab function gm_wlanhdlTimeAndFrequencySynchronization/WLANTimeAndFrequencySynchronization/Coarse Time Sync/Correlator/delayedCorrelation/DTadjust/DTadjust ==
  data: in input; out output; wlanConfig parameter
function out = DTadjust(in,wlanConfig)
%#codegen
if isfloat(in)
    out = in;
else
    WL = in.WordLength;
    FL = WL - (log2(wlanConfig.lstfLen)+1)-1;
    out = fi(in,1,WL,FL);
end

== matlab function gm_wlanhdlTimeAndFrequencySynchronization/WLANTimeAndFrequencySynchronization/Coarse Time Sync/Energy Calculator/magnitudeSquared/MagnitudeSquared/DTadjust/DTadjust ==
  data: in input; out output; wlanConfig parameter
function out = DTadjust(in,wlanConfig)
%#codegen
if isfloat(in)
    out = in;
else
    WL = in.WordLength;
    FL = WL - (log2(wlanConfig.lstfLen)+1)-1;
    out = fi(in,1,WL,FL);
end

== matlab function gm_wlanhdlTimeAndFrequencySynchronization/WLANTimeAndFrequencySynchronization/Fine CFO Estimation and Correction/Fine CFO Estimation/sample FreqOff/Sample FreqOff ==
  data: freqOffIn input; freqOffOut output; enb input; rst input
function freqOffOut = sampleFreqOff(freqOffIn,enb,rst)
%#codegen

persistent freqReg;
persistent freqFlag;

if isempty(freqReg)||rst
    freqReg = cast(0,'like',freqOffIn);
    freqFlag = true;
end

if enb && freqFlag   
        freqReg = freqOffIn;
        freqFlag = false;      
end

freqOffOut = freqReg;

== matlab function gm_wlanhdlTimeAndFrequencySynchronization/WLANTimeAndFrequencySynchronization/Fine Time Sync/Peak Searcher/peakDetector/dataSelector /MATLAB Function1 ==
  data: syncEn input; dataIn input; dataOut output; validIn input
function dataOut = dataSelector(syncEn,dataIn,validIn)
%#codegen

if validIn && syncEn
    dataOut = dataIn;
else
    dataOut = cast(complex(0,0),'like',dataIn);
end

== matlab function gm_wlanhdlTimeAndFrequencySynchronization/WLANTimeAndFrequencySynchronization/Coarse CFO Estimation and Correction/Coarse CFO Estimation/Sample FreqOff/Sample FreqOff ==
  data: freqOffIn input; freqOffOut output; enb input; rst input
function freqOffOut = sampleFreqOff(freqOffIn,enb,rst)
%#codegen

persistent freqReg;
persistent freqFlag;

if isempty(freqReg)||rst
    freqReg = cast(0,'like',freqOffIn);
    freqFlag = true;
end

if enb && freqFlag   
        freqReg = freqOffIn;
        freqFlag = false;      
end

freqOffOut = freqReg;

== matlab function gm_wlanhdlTimeAndFrequencySynchronization/WLANTimeAndFrequencySynchronization/Fine Time Sync/Peak Searcher/maxPeakSearcher/maxPeakSearcher/maxPeakSearcher ==
  data: dataIn input; maxPeak output; validIn input; countValue input; reset input; wlanConfig parameter
function maxPeak  = maxPeakSearcher(dataIn,validIn,countValue,reset,wlanConfig)
%#codegen

persistent maxPeakReg;
persistent maxPeakPrev;
persistent maxValueReg;

if isempty(maxPeakReg) || reset
    maxValueReg = cast(0,'like',dataIn);
    maxPeakReg = cast(0,'like',countValue);
    maxPeakPrev = cast(0,'like',countValue);
end

if validIn
    if dataIn > maxValueReg        
       maxPeakReg = countValue;
       maxValueReg = dataIn;
    end
end

if countValue == 2*wlanConfig.corrLen-1
    maxPeak  = maxPeakReg-wlanConfig.corrLen;
    maxPeakPrev = maxPeak;
else
    maxPeak  = cast(maxPeakPrev,'like',countValue);
end

== matlab function gm_wlanhdlTimeAndFrequencySynchronization/WLANTimeAndFrequencySynchronization/Coarse Time Sync/Energy Calculator/streamSynchronizer/StreamSyncronizer/StreamSyncronizer ==
  data: pop input; dataIn input; dataOut output; push input; validOut output; depth parameter
function [dataOut, validOut] = SynchronousFIFO(pop,dataIn,push,depth)
    %#codegen
    
    coder.extrinsic('warning');
    coder.extrinsic('num2str');
    
    persistent wrAddr rdAddr dataOutReg validOutReg mem level;
    
    %------------------------------------------------------------------------
    % Constants
    %------------------------------------------------------------------------
    
    addrWL = nextpow2(depth);
    
    %------------------------------------------------------------------------
    % Persistent variable initialization
    %------------------------------------------------------------------------
    
    if isempty(mem)
        
        wrAddr      = fi(0,0,addrWL,0,hdlfimath);
        rdAddr      = fi(0,0,addrWL,0,hdlfimath);
        dataOutReg  = cast(0,'like',dataIn);
        validOutReg = false;
        mem         = zeros(depth,1,'like',dataIn);
        % For generating warnings only. Not for code gen.
        level       = int16(0);
                
    end
    
    %------------------------------------------------------------------------
    % Outputs
    %------------------------------------------------------------------------
    
    dataOut  = dataOutReg;
    validOut = validOutReg;
    
    %------------------------------------------------------------------------
    % Calculate next state values
    %------------------------------------------------------------------------
    
    if pop
        
        dataOutReg(:) = mem(rdAddr+1);
        rdAddr(:)     = rdAddr+1;
        level(:)      = level-1;
        
        if level < 0
            warning('Buffer underflow: attempt to pop data out of empty buffer.');
        end
        
    end
    
    if push
        
        mem(wrAddr+1) = dataIn;
        wrAddr(:)     = wrAddr+1;
        level(:)      = level+1;
        
        if level > depth            
            warning(['Buffer overflow: attempt to push data into full buffer. Level = ', num2str(level), '.']);
        end
        
    end
    
    validOutReg = pop;
    
end

== matlab function gm_wlanhdlTimeAndFrequencySynchronization/WLANTimeAndFrequencySynchronization/Coarse Time Sync/Peak Detector/MATLAB Function1/MATLAB Function1 ==
  data: syncEn input; dataIn input; dataOut output; validIn input
function dataOut = dataSelector(syncEn,dataIn,validIn)
%#codegen

if validIn && syncEn
    dataOut = dataIn;
else
    dataOut = cast(complex(0,0),'like',dataIn);
end
